simulink model "Single_phase_Half_wave_uncontrolled_rectifier_RL_Motor_Load"  (R2023b)
settings: Solver=ode23tb  StartTime=0.0  StopTime=0.08  RelTol=1e-3
libraries: spsVoltageMeasurementLib x2, spsDiodeLib x1, spsACVoltageSourceLib x1, spsDCVoltageSourceLib x1, spsSeriesRLCBranchLib x1, spspowerguiLib x1
settings Model: Creator=HP  LastModifiedBy=HP

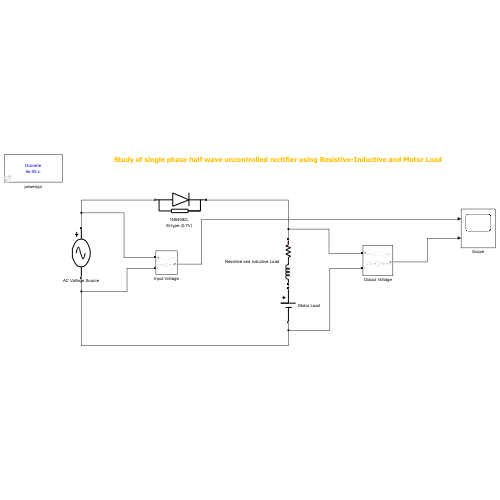
[thumbnail: Simulink's stored preview of the top-level diagram]
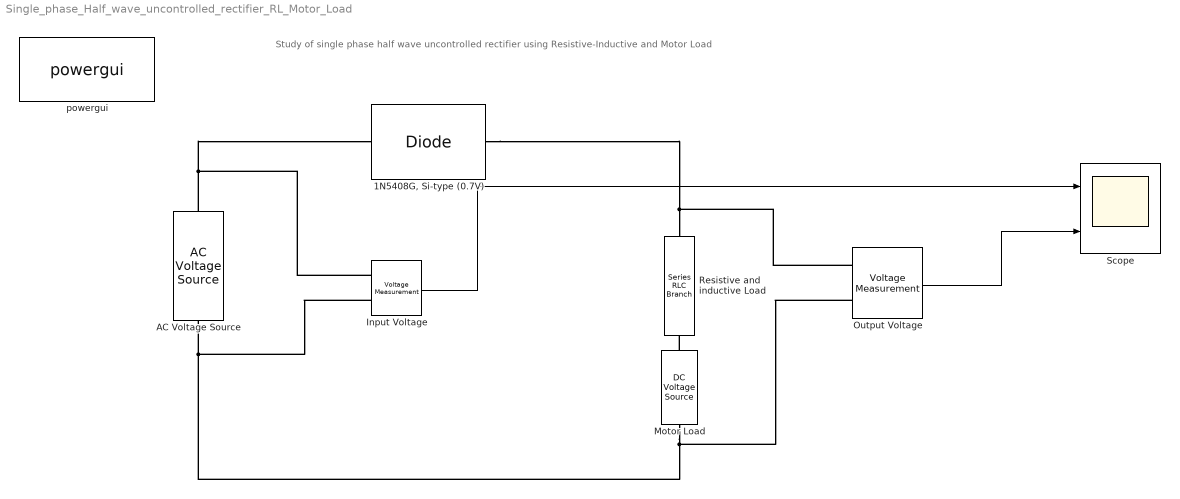
== system Single_phase_Half_wave_uncontrolled_rectifier_RL_Motor_Load ==
  note: Study of single phase half wave uncontrolled rectifier using Resistive-Inductive and Motor Load
  "1N5408G, Si-type (0.7V)  " : spsDiodeLib/Diode  Ron=0.1  Lon=0  Vf=0.7  IC=0  UseSnubber=0  Rs=400  Cs=250e-9  Measurements=off
  AC Voltage Source : spsACVoltageSourceLib/AC Voltage Source  Amplitude=220  Phase=0  Frequency=50  SampleTime=0  Measurements=Voltage  BusType=swing  Pref=10e3  Qref=0  Qmin=-inf  Qmax=+inf
  Input Voltage : spsVoltageMeasurementLib/Voltage Measurement  PhasorSimulation=off  OutputType=Complex  PSBequivalent=0
  Motor Load : spsDCVoltageSourceLib/DC Voltage Source  Amplitude=100  Measurements=None
  Output Voltage : spsVoltageMeasurementLib/Voltage Measurement  PhasorSimulation=off  OutputType=Complex  PSBequivalent=0
  Resistive and inductive Load : spsSeriesRLCBranchLib/Series RLC Branch  LConnTagsString=__new0  RConnTagsString=__new0  BranchType=RL  Resistance=1000  Inductance=0.04  SetiL0=off  InitialCurrent=0  Capacitance=1e-6  Setx0=off  InitialVoltage=0  Measurements=Branch voltage
  Scope : Scope  NumInputPorts=2
  powergui : spspowerguiLib/powergui  Priority=1  SimulationMode=Discrete  SampleTime=50e-6  frequency=60  Iterations=50  frequencyindice=50  Pbase=100e6  ErrMax=1e-4  UnitsV=kV  UnitsW=MW  buscounter=0  FunctionMessages=off  echomessages=off  EnableUseOfTLC=off  CurrentSourceSwitches=off  DisableSnubberDevices=off  DisableRonSwitches=off  DisableVfSwitches=off  DisplayEquations=off  AutomaticDiscreteSolvers=off  SolverType=Tustin/Backward Euler (TBE)  Interpol=off  ExternalGateDelay=off  methode=off  Ts=100  x0status=blocks  SPID=on  SwTol=0  HookPort=off  NonlinearTolerance=1e-4  nMaxIteration=100  ContinueOnMaxIteration=off  RestoreLinks=warning  ResistiveCurrentMeasurement=off  Frange=[0:2:500]  Ylog=off  Xlog=on  ShowGrid=off  save=off  variable=ZData  structure=0  ZoomFFT=off  StartTime=0.0  cycles=1  DisplayStyle=1  fundamental=60  FreqAxis=off  MaxFrequency=1000  frequencyindicesteady=1  RmsSteady=1  display=off
  wires:
  Output Voltage/1 -> Scope/2
  Input Voltage/1 -> Scope/1
  connections:
  AC Voltage Source/RConn1 -- Input Voltage/LConn1 -- "1N5408G, Si-type (0.7V)  "/LConn1
  "1N5408G, Si-type (0.7V)  "/RConn1 -- Resistive and inductive Load/LConn1 -- Output Voltage/LConn1
  Motor Load/RConn1 -- Resistive and inductive Load/RConn1
  Motor Load/LConn1 -- Output Voltage/LConn2 -- Input Voltage/LConn2 -- AC Voltage Source/LConn1
